simulink model "IEEE9Buses"  (R2024b)
settings: Solver=FixedStepAuto  StartTime=0  StopTime=5  FixedStep=1e-6  RelTol=1e-3
values from neighbouring files (symbols this model uses):
  SG_D_1_D = 0.01056    [SG9_parameters.m]
  SG_D_1_EnableSaturation = 0    [SG9_parameters.m]
  SG_D_1_f0 = 60    [SG9_parameters.m]
  SG_D_1_H = 7.5    [SG9_parameters.m]
  SG_D_1_K_A = 20    [SG9_parameters.m]
  SG_D_1_K_E = 1.000000e+1    (= 10)    [SG9_parameters.m]
  SG_D_1_K_F = 2.363    [SG9_parameters.m]
  SG_D_1_K_s = 5    [SG9_parameters.m]
  SG_D_1_R_a = 0.001088    [SG9_parameters.m]
  SG_D_1_S_A = 1    [SG9_parameters.m]
  SG_D_1_S_B = 0.103    [SG9_parameters.m]
  SG_D_1_S_N = 10.659857    [SG9_parameters.m]
  SG_D_1_SpeedPara = 200    [SG9_parameters.m]
  SG_D_1_T_0 = 0.720173    [SG9_parameters.m]
  SG_D_1_T_1 = 0.3    [SG9_parameters.m]
  SG_D_1_T_2 = 0.05    [SG9_parameters.m]
  SG_D_1_T_3 = 0.02    [SG9_parameters.m]
  SG_D_1_T_4 = 0.005    [SG9_parameters.m]
  SG_D_1_T_A = 0.02    [SG9_parameters.m]
  SG_D_1_T_dd = 8.000000e+0    (= 8)    [SG9_parameters.m]
  SG_D_1_T_ddd = 0.04    [SG9_parameters.m]
  SG_D_1_T_E = 0.314    [SG9_parameters.m]
  SG_D_1_T_F = 0.35    [SG9_parameters.m]
  SG_D_1_T_qd = 0.8    [SG9_parameters.m]
  SG_D_1_T_qdd = 0.02    [SG9_parameters.m]
  SG_D_1_T_speed = 0.1    [SG9_parameters.m]
  SG_D_1_T_w = 0.5    [SG9_parameters.m]
  SG_D_1_V_ref = 1.990276    [SG9_parameters.m]
  SG_D_1_w_ref = 376.991118    [SG9_parameters.m]
  SG_D_1_x_d = 1.9    [SG9_parameters.m]
  SG_D_1_x_dd = 0.302    [SG9_parameters.m]
  SG_D_1_x_ddd = 0.204    [SG9_parameters.m]
  SG_D_1_x_l = 0.05    [SG9_parameters.m]
  SG_D_1_x_q = 1.3    [SG9_parameters.m]
  SG_D_1_x_qd = 0.5    [SG9_parameters.m]
  SG_D_1_x_qdd = 0.3    [SG9_parameters.m]
  SG_D_2_D = 0.01056    [SG9_parameters.m]
  SG_D_2_EnableSaturation = 0    [SG9_parameters.m]
  SG_D_2_f0 = 60    [SG9_parameters.m]
  SG_D_2_H = 7.5    [SG9_parameters.m]
  SG_D_2_K_A = 20    [SG9_parameters.m]
  SG_D_2_K_E = 1.000000e+1    (= 10)    [SG9_parameters.m]
  SG_D_2_K_F = 2.363    [SG9_parameters.m]
  SG_D_2_K_s = 0.5    [SG9_parameters.m]
  SG_D_2_R_a = 0.001088    [SG9_parameters.m]
  SG_D_2_S_A = 1    [SG9_parameters.m]
  SG_D_2_S_B = 0.103    [SG9_parameters.m]
  SG_D_2_S_N = 10.659857    [SG9_parameters.m]
  SG_D_2_SpeedPara = 200    [SG9_parameters.m]
  SG_D_2_T_0 = 1.632913    [SG9_parameters.m]
  SG_D_2_T_1 = 0.2    [SG9_parameters.m]
  SG_D_2_T_2 = 0.05    [SG9_parameters.m]
  SG_D_2_T_3 = 0.02    [SG9_parameters.m]
  SG_D_2_T_4 = 0.005    [SG9_parameters.m]
  SG_D_2_T_A = 0.02    [SG9_parameters.m]
  SG_D_2_T_dd = 8.000000e+0    (= 8)    [SG9_parameters.m]
  SG_D_2_T_ddd = 0.04    [SG9_parameters.m]
  SG_D_2_T_E = 0.314    [SG9_parameters.m]
  SG_D_2_T_F = 0.35    [SG9_parameters.m]
  SG_D_2_T_qd = 0.8    [SG9_parameters.m]
  SG_D_2_T_qdd = 0.02    [SG9_parameters.m]
  SG_D_2_T_speed = 0.1    [SG9_parameters.m]
  SG_D_2_T_w = 0.5    [SG9_parameters.m]
  SG_D_2_V_ref = 2.662631    [SG9_parameters.m]
  SG_D_2_w_ref = 376.991118    [SG9_parameters.m]
  SG_D_2_x_d = 1.9    [SG9_parameters.m]
  SG_D_2_x_dd = 0.302    [SG9_parameters.m]
  SG_D_2_x_ddd = 0.204    [SG9_parameters.m]
  SG_D_2_x_l = 0.05    [SG9_parameters.m]
  SG_D_2_x_q = 1.3    [SG9_parameters.m]
  SG_D_2_x_qd = 0.5    [SG9_parameters.m]
  SG_D_2_x_qdd = 0.3    [SG9_parameters.m]
  SG_D_3_D = 0.01056    [SG9_parameters.m]
  SG_D_3_EnableSaturation = 0    [SG9_parameters.m]
  SG_D_3_f0 = 60    [SG9_parameters.m]
  SG_D_3_H = 7.5    [SG9_parameters.m]
  SG_D_3_K_A = 20    [SG9_parameters.m]
  SG_D_3_K_E = 1.000000e+1    (= 10)    [SG9_parameters.m]
  SG_D_3_K_F = 2.363    [SG9_parameters.m]
  SG_D_3_K_s = 0.5    [SG9_parameters.m]
  SG_D_3_R_a = 0.001088    [SG9_parameters.m]
  SG_D_3_S_A = 1    [SG9_parameters.m]
  SG_D_3_S_B = 0.103    [SG9_parameters.m]
  SG_D_3_S_N = 10.659857    [SG9_parameters.m]
  SG_D_3_SpeedPara = 200    [SG9_parameters.m]
  SG_D_3_T_0 = 0.850788    [SG9_parameters.m]
  SG_D_3_T_1 = 0.2    [SG9_parameters.m]
  SG_D_3_T_2 = 0.05    [SG9_parameters.m]
  SG_D_3_T_3 = 0.02    [SG9_parameters.m]
  SG_D_3_T_4 = 0.005    [SG9_parameters.m]
  SG_D_3_T_A = 0.02    [SG9_parameters.m]
  SG_D_3_T_dd = 8.000000e+0    (= 8)    [SG9_parameters.m]
  SG_D_3_T_ddd = 0.04    [SG9_parameters.m]
  SG_D_3_T_E = 0.314    [SG9_parameters.m]
  SG_D_3_T_F = 0.35    [SG9_parameters.m]
  SG_D_3_T_qd = 0.8    [SG9_parameters.m]
  SG_D_3_T_qdd = 0.02    [SG9_parameters.m]
  SG_D_3_T_speed = 0.1    [SG9_parameters.m]
  SG_D_3_T_w = 0.5    [SG9_parameters.m]
  SG_D_3_V_ref = 1.915682    [SG9_parameters.m]
  SG_D_3_w_ref = 376.991118    [SG9_parameters.m]
  SG_D_3_x_d = 1.9    [SG9_parameters.m]
  SG_D_3_x_dd = 0.302    [SG9_parameters.m]
  SG_D_3_x_ddd = 0.204    [SG9_parameters.m]
  SG_D_3_x_l = 0.05    [SG9_parameters.m]
  SG_D_3_x_q = 1.3    [SG9_parameters.m]
  SG_D_3_x_qd = 0.5    [SG9_parameters.m]
  SG_D_3_x_qdd = 0.3    [SG9_parameters.m]
(part 8 of 9)

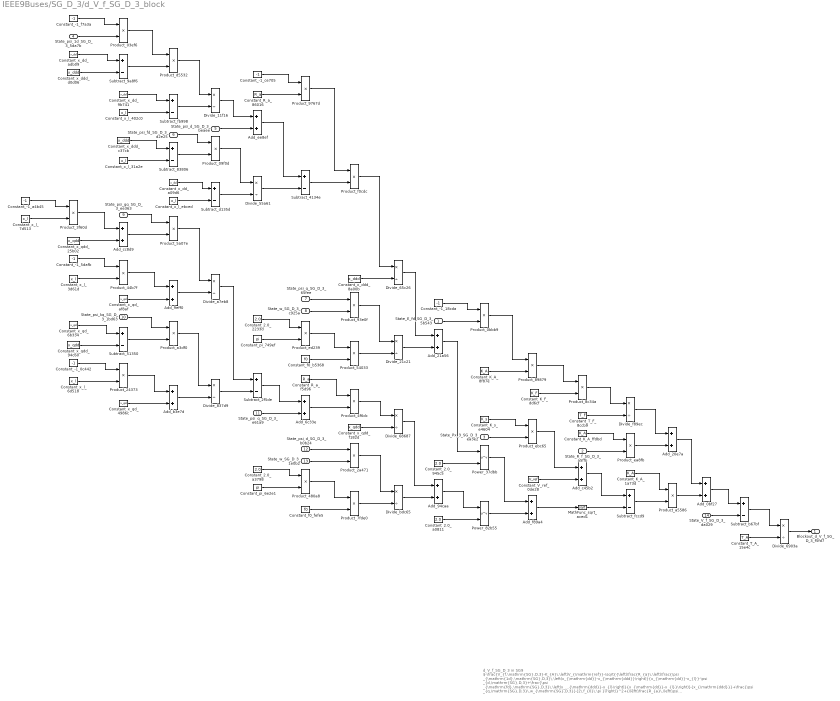
== system IEEE9Buses/SG_D_3/d_V_f_SG_D_3_block ==
  note: d_V_f_SG_D_3 in SG9
      | $-\frac{V_{f,\mathrm{SG},D,3}-K_{A}\,\left(V_{\mathrm{ref}}-\sqrt{{\left(\frac{R_{a}\,\left(\frac{\psi _{\mathrm{1d},\mathrm{SG},D,3}\,\left(x_{\mathrm{dd}}-x_{\mathrm{ddd}}\right)}{x_{\mathrm{dd}}-x_{l}}-\psi _{d,\mathrm{SG},D,3}+\frac{\psi _{\mathrm{fd},\mathrm{SG},D,3}\,\left(x_{\mathrm{ddd}}-x_{l}\right)}{x_{\mathrm{dd}}-x_{l}}\right)}{x_{\mathrm{ddd}}}+\frac{\psi _{q,\mathrm{SG},D,3}\,w_{\mathrm{SG},D,3}}{2\,f_{0}\,\pi }\right)}^2+{\left(\frac{R_{a}\,\left(\psi _{q,\mathrm{SG},D,3}+\frac{\psi _{\mathrm{gq},\mathrm{SG},D,3}\,\left(x_{l}-x_{\mathrm{qdd}}\right)}{x_{l}-x_{\mathrm{qd}}}+\frac{\psi _{\mathrm{kq},\mathrm{SG},D,3}\,\left(x_{\mathrm{qd}}-x_{\mathrm{qdd}}\right)}{x_{l}-x_{\mathrm{qd}}}\right)}{x_{\mathrm{qdd}}}+\frac{\psi _{d,\mathrm{SG},D,3}\,w_{\mathrm{SG},D,3}}{2\,f_{0}\,\pi }\right)}^2}+K_{s}\,\mathrm{Px}_{3,\mathrm{SG},D,3}\right)-K_{A}\,R_{f,\mathrm{SG},D,3}+\frac{E_{\mathrm{fd},\mathrm{SG},D,3}\,K_{A}\,K_{F}}{T_{F}}}{T_{A}}$
      | Automatically generated on 2025-09-12 21:33:42 .
  State_E_fd_SG_D_3_5b543 : Inport
  State_R_f_SG_D_3_a5ffb : Inport  Port=2
  State_Px_3_SG_D_3_ea3e2 : Inport  Port=3
  State_psi_1d_SG_D_3_5da7b : Inport  Port=4
  State_psi_d_SG_D_3_beaee : Inport  Port=5
  State_psi_fd_SG_D_3_d2e25 : Inport  Port=6
  State_psi_q_SG_D_3_65fee : Inport  Port=7
  State_w_SG_D_3_c925a : Inport  Port=8
  State_psi_gq_SG_D_3_ee363 : Inport  Port=9
  State_psi_kq_SG_D_3_1bd63 : Inport  Port=10
  State_psi_q_SG_D_3_e61a9 : Inport  Port=11
  State_psi_d_SG_D_3_b0b24 : Inport  Port=12
  State_w_SG_D_3_1e0b2 : Inport  Port=13
  State_V_f_SG_D_3_da029 : Inport  Port=14
  Add_0bf27 : Sum
  Add_20e7a : Sum
  Add_21a56 : Sum
  Add_6c33e : Sum
  Add_94caa : Sum
  Add_9eff0 : Sum
  Add_b3e7d : Sum
  Add_c45b2 : Sum
  Add_cc8d9 : Sum
  Add_ee8ef : Sum
  Add_f89a4 : Sum
  Constant_-1_0c442 : Constant  Value=-1
  Constant_-1_18cda : Constant  Value=-1
  Constant_-1_5dafb : Constant  Value=-1
  Constant_-1_a4b45 : Constant  Value=-1
  Constant_-1_ce705 : Constant  Value=-1
  Constant_-1_f7a3a : Constant  Value=-1
  Constant_2.0_2233d : Constant  Value=2.0
  Constant_2.0_945c5 : Constant  Value=2.0
  Constant_2.0_a0811 : Constant  Value=2.0
  Constant_2.0_a3798 : Constant  Value=2.0
  Constant_K_A_1a73d : Constant  Value=K_A
  Constant_K_A_8f87e : Constant  Value=K_A
  Constant_K_A_ffdbd : Constant  Value=K_A
  Constant_K_F_dd6cf : Constant  Value=K_F
  Constant_K_s_e4604 : Constant  Value=K_s
  Constant_R_a_86016 : Constant  Value=R_a
  Constant_R_a_f5d96 : Constant  Value=R_a
  Constant_T_A_15e4c : Constant  Value=T_A
  Constant_T_F_8ccb9 : Constant  Value=T_F
  Constant_V_ref_0de28 : Constant  Value=V_ref
  Constant_f0_b5368 : Constant  Value=f0
  Constant_f0_fefe5 : Constant  Value=f0
  Constant_pi_6e2e1 : Constant  Value=pi
  Constant_pi_749ef : Constant  Value=pi
  Constant_x_dd_9b741 : Constant  Value=x_dd
  Constant_x_dd_a09d6 : Constant  Value=x_dd
  Constant_x_dd_adb09 : Constant  Value=x_dd
  Constant_x_ddd_8a00b : Constant  Value=x_ddd
  Constant_x_ddd_c37cb : Constant  Value=x_ddd
  Constant_x_ddd_d0d06 : Constant  Value=x_ddd
  Constant_x_l_31a2e : Constant  Value=x_l
  Constant_x_l_3d61d : Constant  Value=x_l
  Constant_x_l_402c0 : Constant  Value=x_l
  Constant_x_l_6d518 : Constant  Value=x_l
  Constant_x_l_7d513 : Constant  Value=x_l
  Constant_x_l_ebced : Constant  Value=x_l
  Constant_x_qd_4986c : Constant  Value=x_qd
  Constant_x_qd_6b334 : Constant  Value=x_qd
  Constant_x_qd_af8af : Constant  Value=x_qd
  Constant_x_qdd_25b02 : Constant  Value=x_qdd
  Constant_x_qdd_94c60 : Constant  Value=x_qdd
  Constant_x_qdd_f182d : Constant  Value=x_qdd
  Divide_11f16 : Product  Inputs=*/
  Divide_21c21 : Product  Inputs=*/
  Divide_55a61 : Product  Inputs=*/
  Divide_65c26 : Product  Inputs=*/
  Divide_68687 : Product  Inputs=*/
  Divide_6903a : Product  Inputs=*/
  Divide_837d9 : Product  Inputs=*/
  Divide_a7eb8 : Product  Inputs=*/
  Divide_bdc65 : Product  Inputs=*/
  Divide_f89ec : Product  Inputs=*/
  MathFunc_sqrt_aced1 : Sqrt
  Power_37dbb : Math  Operator=pow
  Power_82b55 : Math  Operator=pow
  Product_03ef6 : Product
  Product_09f0d : Product
  Product_0bbb9 : Product
  Product_24373 : Product
  Product_2a471 : Product
  Product_3f60d : Product
  Product_44b7f : Product
  Product_480a8 : Product
  Product_4f6dc : Product
  Product_54033 : Product
  Product_5a07e : Product
  Product_7fde0 : Product
  Product_89879 : Product
  Product_8c34a : Product
  Product_93e0f : Product
  Product_9767d : Product
  Product_a3df0 : Product
  Product_a5586 : Product
  Product_d5532 : Product
  Product_ea8fb : Product
  Product_ebc65 : Product
  Product_ed239 : Product
  Product_f0cdc : Product
  Subtract_2f5de : Sum  Inputs=+-
  Subtract_4134e : Sum  Inputs=+-
  Subtract_51350 : Sum  Inputs=+-
  Subtract_83806 : Sum  Inputs=+-
  Subtract_9a8f6 : Sum  Inputs=+-
  Subtract_b67bf : Sum  Inputs=+-
  Subtract_d135d : Sum  Inputs=+-
  Subtract_fb998 : Sum  Inputs=+-
  Subtract_fccd9 : Sum  Inputs=+-
  Blockout_d_V_f_SG_D_3_f5fd7 : Outport
  wires:
  Constant_K_A_ffdbd/1 -> Product_ea8fb/1
  Constant_-1_a4b45/1 -> Product_3f60d/1
  Subtract_83806/1 -> Product_09f0d/2
  Constant_x_l_7d513/1 -> Product_3f60d/2
  Divide_bdc65/1 -> Add_94caa/2
  Constant_-1_f7a3a/1 -> Product_03ef6/1
  State_psi_1d_SG_D_3_5da7b/1 -> Product_03ef6/2
  Constant_x_dd_adb09/1 -> Subtract_9a8f6/1
  Divide_55a61/1 -> Subtract_4134e/2
  Product_3f60d/1 -> Add_cc8d9/1
  Constant_x_qdd_25b02/1 -> Add_cc8d9/2
  Constant_x_ddd_d0d06/1 -> Subtract_9a8f6/2
  Constant_2.0_a0811/1 -> Power_82b55/2
  Constant_-1_5dafb/1 -> Product_44b7f/1
  Divide_a7eb8/1 -> Subtract_2f5de/1
  Subtract_fb998/1 -> Divide_11f16/2
  Constant_x_l_3d61d/1 -> Product_44b7f/2
  Constant_x_qd_6b334/1 -> Subtract_51350/1
  State_w_SG_D_3_c925a/1 -> Product_93e0f/2
  Constant_x_qdd_94c60/1 -> Subtract_51350/2
  Constant_2.0_2233d/1 -> Product_ed239/1
  Constant_-1_0c442/1 -> Product_24373/1
  Constant_pi_749ef/1 -> Product_ed239/2
  Add_ee8ef/1 -> Subtract_4134e/1
  Constant_x_l_6d518/1 -> Product_24373/2
  Product_03ef6/1 -> Product_d5532/1
  Subtract_9a8f6/1 -> Product_d5532/2
  Constant_2.0_a3798/1 -> Product_480a8/1
  Constant_x_dd_9b741/1 -> Subtract_fb998/1
  Constant_pi_6e2e1/1 -> Product_480a8/2
  Constant_x_l_402c0/1 -> Subtract_fb998/2
  Constant_x_ddd_c37cb/1 -> Subtract_83806/1
  Constant_x_l_31a2e/1 -> Subtract_83806/2
  State_psi_gq_SG_D_3_ee363/1 -> Product_5a07e/1
  Constant_x_l_ebced/1 -> Subtract_d135d/2
  Add_cc8d9/1 -> Product_5a07e/2
  Product_44b7f/1 -> Add_9eff0/1
  Product_5a07e/1 -> Divide_a7eb8/1
  Constant_x_qd_af8af/1 -> Add_9eff0/2
  State_psi_kq_SG_D_3_1bd63/1 -> Product_a3df0/1
  State_psi_q_SG_D_3_65fee/1 -> Product_93e0f/1
  Add_21a56/1 -> Power_37dbb/1
  Subtract_51350/1 -> Product_a3df0/2
  Constant_f0_b5368/1 -> Product_54033/2
  Product_ed239/1 -> Product_54033/1
  Constant_x_qd_4986c/1 -> Add_b3e7d/2
  Product_24373/1 -> Add_b3e7d/1
  Product_d5532/1 -> Divide_11f16/1
  State_psi_fd_SG_D_3_d2e25/1 -> Product_09f0d/1
  Constant_x_dd_a09d6/1 -> Subtract_d135d/1
  Add_9eff0/1 -> Divide_a7eb8/2
  Add_f89a4/1 -> MathFunc_sqrt_aced1/1
  Product_a3df0/1 -> Divide_837d9/1
  Add_b3e7d/1 -> Divide_837d9/2
  Product_9767d/1 -> Product_f0cdc/1
  Divide_11f16/1 -> Add_ee8ef/1
  Add_c45b2/1 -> Subtract_fccd9/1
  State_psi_d_SG_D_3_beaee/1 -> Add_ee8ef/2
  Product_09f0d/1 -> Divide_55a61/1
  Subtract_d135d/1 -> Divide_55a61/2
  MathFunc_sqrt_aced1/1 -> Subtract_fccd9/2
  Divide_837d9/1 -> Subtract_2f5de/2
  Constant_-1_ce705/1 -> Product_9767d/1
  Constant_R_a_86016/1 -> Product_9767d/2
  Subtract_2f5de/1 -> Add_6c33e/1
  State_psi_q_SG_D_3_e61a9/1 -> Add_6c33e/2
  Subtract_4134e/1 -> Product_f0cdc/2
  Constant_R_a_f5d96/1 -> Product_4f6dc/1
  Add_6c33e/1 -> Product_4f6dc/2
  State_psi_d_SG_D_3_b0b24/1 -> Product_2a471/1
  State_w_SG_D_3_1e0b2/1 -> Product_2a471/2
  Product_480a8/1 -> Product_7fde0/1
  Constant_f0_fefe5/1 -> Product_7fde0/2
  Product_f0cdc/1 -> Divide_65c26/1
  Constant_x_ddd_8a00b/1 -> Divide_65c26/2
  Product_93e0f/1 -> Divide_21c21/1
  Product_54033/1 -> Divide_21c21/2
  Product_4f6dc/1 -> Divide_68687/1
  Constant_x_qdd_f182d/1 -> Divide_68687/2
  Product_2a471/1 -> Divide_bdc65/1
  Product_7fde0/1 -> Divide_bdc65/2
  Divide_65c26/1 -> Add_21a56/1
  Divide_21c21/1 -> Add_21a56/2
  Divide_68687/1 -> Add_94caa/1
  Constant_-1_18cda/1 -> Product_0bbb9/1
  State_E_fd_SG_D_3_5b543/1 -> Product_0bbb9/2
  Constant_2.0_945c5/1 -> Power_37dbb/2
  Add_94caa/1 -> Power_82b55/1
  Product_0bbb9/1 -> Product_89879/1
  Constant_K_A_8f87e/1 -> Product_89879/2
  Constant_K_s_e4604/1 -> Product_ebc65/1
  State_Px_3_SG_D_3_ea3e2/1 -> Product_ebc65/2
  Power_37dbb/1 -> Add_f89a4/1
  Power_82b55/1 -> Add_f89a4/2
  Product_89879/1 -> Product_8c34a/1
  Constant_K_F_dd6cf/1 -> Product_8c34a/2
  Product_ebc65/1 -> Add_c45b2/1
  Constant_V_ref_0de28/1 -> Add_c45b2/2
  Product_8c34a/1 -> Divide_f89ec/1
  Constant_T_F_8ccb9/1 -> Divide_f89ec/2
  Add_0bf27/1 -> Subtract_b67bf/1
  State_R_f_SG_D_3_a5ffb/1 -> Product_ea8fb/2
  Divide_f89ec/1 -> Add_20e7a/1
  Product_ea8fb/1 -> Add_20e7a/2
  Constant_K_A_1a73d/1 -> Product_a5586/1
  Subtract_fccd9/1 -> Product_a5586/2
  Add_20e7a/1 -> Add_0bf27/1
  Product_a5586/1 -> Add_0bf27/2
  State_V_f_SG_D_3_da029/1 -> Subtract_b67bf/2
  Subtract_b67bf/1 -> Divide_6903a/1
  Constant_T_A_15e4c/1 -> Divide_6903a/2
  Divide_6903a/1 -> Blockout_d_V_f_SG_D_3_f5fd7/1

== system IEEE9Buses/SG_D_3/d_psi_1d_SG_D_3_block ==
  note: d_psi_1d_SG_D_3 in SG9
      | $-\frac{\psi _{\mathrm{1d},\mathrm{SG},D,3}-\psi _{\mathrm{fd},\mathrm{SG},D,3}+\frac{\left(x_{\mathrm{dd}}-x_{l}\right)\,\left(\frac{\psi _{\mathrm{1d},\mathrm{SG},D,3}\,\left(x_{\mathrm{dd}}-x_{\mathrm{ddd}}\right)}{x_{\mathrm{dd}}-x_{l}}-\psi _{d,\mathrm{SG},D,3}+\frac{\psi _{\mathrm{fd},\mathrm{SG},D,3}\,\left(x_{\mathrm{ddd}}-x_{l}\right)}{x_{\mathrm{dd}}-x_{l}}\right)}{x_{\mathrm{ddd}}}}{T_{\mathrm{ddd}}}$
      | Automatically generated on 2025-09-12 21:33:17 .
  State_psi_1d_SG_D_3_400ff : Inport
  State_psi_fd_SG_D_3_31a8d : Inport  Port=2
  State_psi_1d_SG_D_3_f2eaa : Inport  Port=3
  State_psi_d_SG_D_3_c9b51 : Inport  Port=4
  State_psi_fd_SG_D_3_47081 : Inport  Port=5
  Add_42e95 : Sum
  Add_4c52e : Sum
  Add_9e772 : Sum
  Constant_-1_54a57 : Constant  Value=-1
  Constant_-1_6696c : Constant  Value=-1
  Constant_T_ddd_7d9a7 : Constant  Value=T_ddd
  Constant_x_dd_313f0 : Constant  Value=x_dd
  Constant_x_dd_447e3 : Constant  Value=x_dd
  Constant_x_dd_5a1d4 : Constant  Value=x_dd
  Constant_x_dd_6452b : Constant  Value=x_dd
  Constant_x_ddd_d782d : Constant  Value=x_ddd
  Constant_x_ddd_f181f : Constant  Value=x_ddd
  Constant_x_ddd_f90f1 : Constant  Value=x_ddd
  Constant_x_l_03c08 : Constant  Value=x_l
  Constant_x_l_57332 : Constant  Value=x_l
  Constant_x_l_6982e : Constant  Value=x_l
  Constant_x_l_f8376 : Constant  Value=x_l
  Divide_209ea : Product  Inputs=*/
  Divide_21392 : Product  Inputs=*/
  Divide_56b1a : Product  Inputs=*/
  Divide_59c36 : Product  Inputs=*/
  Product_2f78e : Product
  Product_628a4 : Product
  Product_9daab : Product
  Product_a8839 : Product
  Product_cc23d : Product
  Subtract_222c1 : Sum  Inputs=+-
  Subtract_2de3d : Sum  Inputs=+-
  Subtract_d21cf : Sum  Inputs=+-
  Subtract_d485e : Sum  Inputs=+-
  Subtract_d4c0d : Sum  Inputs=+-
  Subtract_f157f : Sum  Inputs=+-
  Blockout_d_psi_1d_SG_D_3_883d4 : Outport
  wires:
  Divide_59c36/1 -> Add_4c52e/1
  Subtract_222c1/1 -> Product_a8839/2
  Constant_-1_54a57/1 -> Product_9daab/1
  Constant_x_dd_5a1d4/1 -> Subtract_d4c0d/1
  State_psi_1d_SG_D_3_f2eaa/1 -> Product_9daab/2
  Product_9daab/1 -> Product_a8839/1
  Constant_x_dd_447e3/1 -> Subtract_222c1/1
  Constant_x_ddd_f90f1/1 -> Subtract_222c1/2
  Constant_x_l_6982e/1 -> Subtract_d4c0d/2
  Constant_x_ddd_d782d/1 -> Subtract_d485e/1
  Divide_209ea/1 -> Blockout_d_psi_1d_SG_D_3_883d4/1
  Constant_x_l_57332/1 -> Subtract_d485e/2
  Product_a8839/1 -> Divide_59c36/1
  Subtract_d4c0d/1 -> Divide_59c36/2
  State_psi_fd_SG_D_3_47081/1 -> Product_2f78e/1
  Subtract_d485e/1 -> Product_2f78e/2
  Constant_x_dd_313f0/1 -> Subtract_d21cf/1
  Constant_x_l_03c08/1 -> Subtract_d21cf/2
  State_psi_d_SG_D_3_c9b51/1 -> Add_4c52e/2
  Product_2f78e/1 -> Divide_21392/1
  Subtract_d21cf/1 -> Divide_21392/2
  Constant_x_dd_6452b/1 -> Subtract_f157f/1
  Constant_x_l_f8376/1 -> Subtract_f157f/2
  Add_4c52e/1 -> Subtract_2de3d/1
  Divide_21392/1 -> Subtract_2de3d/2
  Constant_-1_6696c/1 -> Product_628a4/1
  State_psi_1d_SG_D_3_400ff/1 -> Product_628a4/2
  State_psi_fd_SG_D_3_31a8d/1 -> Add_42e95/2
  Subtract_f157f/1 -> Product_cc23d/1
  Subtract_2de3d/1 -> Product_cc23d/2
  Product_628a4/1 -> Add_42e95/1
  Product_cc23d/1 -> Divide_56b1a/1
  Constant_x_ddd_f181f/1 -> Divide_56b1a/2
  Add_42e95/1 -> Add_9e772/1
  Divide_56b1a/1 -> Add_9e772/2
  Add_9e772/1 -> Divide_209ea/1
  Constant_T_ddd_7d9a7/1 -> Divide_209ea/2

== system IEEE9Buses/SG_D_3/d_psi_d_SG_D_3_block ==
  note: d_psi_d_SG_D_3 in SG9
      | $2\,\pi \,f_{0}\,\left(v_{d,\mathrm{SG},D,3}\,\sin\left(\theta _{\mathrm{SG},D,3}\right)-v_{q,\mathrm{SG},D,3}\,\cos\left(\theta _{\mathrm{SG},D,3}\right)+\frac{R_{a}\,\left(\frac{\psi _{\mathrm{1d},\mathrm{SG},D,3}\,\left(x_{\mathrm{dd}}-x_{\mathrm{ddd}}\right)}{x_{\mathrm{dd}}-x_{l}}-\psi _{d,\mathrm{SG},D,3}+\frac{\psi _{\mathrm{fd},\mathrm{SG},D,3}\,\left(x_{\mathrm{ddd}}-x_{l}\right)}{x_{\mathrm{dd}}-x_{l}}\right)}{x_{\mathrm{ddd}}}+\frac{\psi _{q,\mathrm{SG},D,3}\,w_{\mathrm{SG},D,3}}{2\,f_{0}\,\pi }\right)$
      | Automatically generated on 2025-09-12 21:33:05 .
  State_psi_1d_SG_D_3_df20d : Inport
  State_psi_d_SG_D_3_5cf2c : Inport  Port=2
  State_psi_fd_SG_D_3_e8974 : Inport  Port=3
  Input_v_d_SG_D_3_a409b : Inport  Port=4
  State_theta_SG_D_3_fa0de : Inport  Port=5
  Input_v_q_SG_D_3_73a19 : Inport  Port=6
  State_theta_SG_D_3_450d2 : Inport  Port=7
  State_psi_q_SG_D_3_3cdee : Inport  Port=8
  State_w_SG_D_3_3c685 : Inport  Port=9
  Add_4bd27 : Sum
  Add_a9d77 : Sum
  Constant_-1_956ee : Constant  Value=-1
  Constant_-2.0_730ca : Constant  Value=-2.0
  Constant_2.0_7512b : Constant  Value=2.0
  Constant_R_a_2c184 : Constant  Value=R_a
  Constant_f0_5f857 : Constant  Value=f0
  Constant_f0_a215f : Constant  Value=f0
  Constant_pi_2d0c1 : Constant  Value=pi
  Constant_pi_a1e68 : Constant  Value=pi
  Constant_x_dd_29953 : Constant  Value=x_dd
  Constant_x_dd_be334 : Constant  Value=x_dd
  Constant_x_dd_bf9bd : Constant  Value=x_dd
  Constant_x_ddd_58709 : Constant  Value=x_ddd
  Constant_x_ddd_84af1 : Constant  Value=x_ddd
  Constant_x_ddd_f35e7 : Constant  Value=x_ddd
  Constant_x_l_06f8d : Constant  Value=x_l
  Constant_x_l_781b5 : Constant  Value=x_l
  Constant_x_l_81dc9 : Constant  Value=x_l
  Divide_3a0c2 : Product  Inputs=*/
  Divide_8a45c : Product  Inputs=*/
  Divide_eab3b : Product  Inputs=*/
  Divide_fffea : Product  Inputs=*/
  MathFunc_cos_6cb2b : Trigonometry  Operator=cos
  MathFunc_sin_c609b : Trigonometry
  Product_075f4 : Product
  Product_1f547 : Product
  Product_53eb6 : Product
  Product_5c8ff : Product
  Product_865d8 : Product
  Product_8be05 : Product
  Product_a313a : Product
  Product_a5a4e : Product
  Product_bb93c : Product
  Product_cddda : Product
  Product_e0659 : Product
  Product_eda06 : Product
  Subtract_46059 : Sum  Inputs=+-
  Subtract_672d9 : Sum  Inputs=+-
  Subtract_6feec : Sum  Inputs=+-
  Subtract_76533 : Sum  Inputs=+-
  Subtract_9ad1c : Sum  Inputs=+-
  Subtract_9d906 : Sum  Inputs=+-
  Subtract_f1390 : Sum  Inputs=+-
  Blockout_d_psi_d_SG_D_3_6cd1a : Outport
  wires:
  Constant_-1_956ee/1 -> Product_a313a/1
  Constant_2.0_7512b/1 -> Product_865d8/1
  Constant_x_dd_bf9bd/1 -> Subtract_f1390/1
  State_psi_1d_SG_D_3_df20d/1 -> Product_a313a/2
  Constant_x_dd_be334/1 -> Subtract_9d906/1
  Constant_pi_a1e68/1 -> Product_865d8/2
  Constant_x_ddd_84af1/1 -> Subtract_f1390/2
  Product_a313a/1 -> Product_e0659/1
  Product_865d8/1 -> Product_8be05/1
  Subtract_f1390/1 -> Product_e0659/2
  Constant_-2.0_730ca/1 -> Product_eda06/1
  Constant_x_l_06f8d/1 -> Subtract_9d906/2
  Constant_x_ddd_58709/1 -> Subtract_9ad1c/1
  Constant_pi_2d0c1/1 -> Product_eda06/2
  Constant_x_l_781b5/1 -> Subtract_9ad1c/2
  Product_bb93c/1 -> Divide_8a45c/1
  Product_e0659/1 -> Divide_fffea/1
  Subtract_9d906/1 -> Divide_fffea/2
  State_psi_fd_SG_D_3_e8974/1 -> Product_5c8ff/1
  Subtract_9ad1c/1 -> Product_5c8ff/2
  Constant_x_dd_29953/1 -> Subtract_46059/1
  Constant_x_l_81dc9/1 -> Subtract_46059/2
  Divide_8a45c/1 -> Subtract_672d9/2
  Divide_fffea/1 -> Add_4bd27/1
  Subtract_6feec/1 -> Product_075f4/2
  State_psi_d_SG_D_3_5cf2c/1 -> Add_4bd27/2
  Product_5c8ff/1 -> Divide_eab3b/1
  Subtract_46059/1 -> Divide_eab3b/2
  Add_4bd27/1 -> Subtract_6feec/1
  Divide_eab3b/1 -> Subtract_6feec/2
  Product_a5a4e/1 -> Add_a9d77/2
  Constant_R_a_2c184/1 -> Product_075f4/1
  Product_53eb6/1 -> Product_cddda/1
  State_theta_SG_D_3_fa0de/1 -> MathFunc_sin_c609b/1
  Product_075f4/1 -> Divide_3a0c2/1
  Constant_x_ddd_f35e7/1 -> Divide_3a0c2/2
  Input_v_d_SG_D_3_a409b/1 -> Product_1f547/1
  State_w_SG_D_3_3c685/1 -> Product_bb93c/2
  MathFunc_sin_c609b/1 -> Product_1f547/2
  State_theta_SG_D_3_450d2/1 -> MathFunc_cos_6cb2b/1
  MathFunc_cos_6cb2b/1 -> Product_a5a4e/2
  Divide_3a0c2/1 -> Subtract_76533/1
  Product_1f547/1 -> Subtract_76533/2
  Input_v_q_SG_D_3_73a19/1 -> Product_a5a4e/1
  State_psi_q_SG_D_3_3cdee/1 -> Product_bb93c/1
  Constant_f0_a215f/1 -> Product_8be05/2
  Subtract_76533/1 -> Add_a9d77/1
  Product_8be05/1 -> Divide_8a45c/2
  Product_eda06/1 -> Product_53eb6/1
  Constant_f0_5f857/1 -> Product_53eb6/2
  Add_a9d77/1 -> Subtract_672d9/1
  Subtract_672d9/1 -> Product_cddda/2
  Product_cddda/1 -> Blockout_d_psi_d_SG_D_3_6cd1a/1

== system IEEE9Buses/SG_D_3/d_psi_fd_SG_D_3_block ==
  note: d_psi_fd_SG_D_3 in SG9
      | $-\frac{\psi _{\mathrm{fd},\mathrm{SG},D,3}-E_{\mathrm{fd},\mathrm{SG},D,3}+\left(x_{d}-x_{\mathrm{dd}}\right)\,\left(\frac{\frac{\psi _{\mathrm{1d},\mathrm{SG},D,3}\,\left(x_{\mathrm{dd}}-x_{\mathrm{ddd}}\right)}{x_{\mathrm{dd}}-x_{l}}-\psi _{d,\mathrm{SG},D,3}+\frac{\psi _{\mathrm{fd},\mathrm{SG},D,3}\,\left(x_{\mathrm{ddd}}-x_{l}\right)}{x_{\mathrm{dd}}-x_{l}}}{x_{\mathrm{ddd}}}-\frac{\left(x_{\mathrm{dd}}-x_{\mathrm{ddd}}\right)\,\left(\psi _{\mathrm{1d},\mathrm{SG},D,3}-\psi _{\mathrm{fd},\mathrm{SG},D,3}+\frac{\left(x_{\mathrm{dd}}-x_{l}\right)\,\left(\frac{\psi _{\mathrm{1d},\mathrm{SG},D,3}\,\left(x_{\mathrm{dd}}-x_{\mathrm{ddd}}\right)}{x_{\mathrm{dd}}-x_{l}}-\psi _{d,\mathrm{SG},D,3}+\frac{\psi _{\mathrm{fd},\mathrm{SG},D,3}\,\left(x_{\mathrm{ddd}}-x_{l}\right)}{x_{\mathrm{dd}}-x_{l}}\right)}{x_{\mathrm{ddd}}}\right)}{{\left(x_{\mathrm{dd}}-x_{l}\right)}^2}\right)}{T_{\mathrm{dd}}}$
      | Automatically generated on 2025-09-12 21:33:14 .
  State_E_fd_SG_D_3_2d5b6 : Inport
  State_psi_fd_SG_D_3_8c274 : Inport  Port=2
  State_psi_1d_SG_D_3_ced24 : Inport  Port=3
  State_psi_fd_SG_D_3_4a37b : Inport  Port=4
  State_psi_1d_SG_D_3_58f7d : Inport  Port=5
  State_psi_d_SG_D_3_264cd : Inport  Port=6
  State_psi_fd_SG_D_3_d3958 : Inport  Port=7
  State_psi_1d_SG_D_3_6cc6d : Inport  Port=8
  State_psi_d_SG_D_3_3305b : Inport  Port=9
  State_psi_fd_SG_D_3_265a7 : Inport  Port=10
  Add_315d4 : Sum
  Add_a78bb : Sum
  Constant_-1_2d1a2 : Constant  Value=-1
  Constant_-1_a4354 : Constant  Value=-1
  Constant_-1_b314b : Constant  Value=-1
  Constant_2.0_a7a8d : Constant  Value=2.0
  Constant_T_dd_9c02c : Constant  Value=T_dd
  Constant_x_d_df3b7 : Constant  Value=x_d
  Constant_x_dd_05d1b : Constant  Value=x_dd
  Constant_x_dd_0c92f : Constant  Value=x_dd
  Constant_x_dd_15bda : Constant  Value=x_dd
  Constant_x_dd_2465f : Constant  Value=x_dd
  Constant_x_dd_5b54a : Constant  Value=x_dd
  Constant_x_dd_8d7a4 : Constant  Value=x_dd
  Constant_x_dd_a5419 : Constant  Value=x_dd
  Constant_x_dd_daca3 : Constant  Value=x_dd
  Constant_x_dd_e1b8f : Constant  Value=x_dd
  Constant_x_dd_ee6c4 : Constant  Value=x_dd
  Constant_x_ddd_4286f : Constant  Value=x_ddd
  Constant_x_ddd_71c11 : Constant  Value=x_ddd
  Constant_x_ddd_a541b : Constant  Value=x_ddd
  Constant_x_ddd_b4a45 : Constant  Value=x_ddd
  Constant_x_ddd_dc6f5 : Constant  Value=x_ddd
  Constant_x_ddd_df8f7 : Constant  Value=x_ddd
  Constant_x_ddd_e0756 : Constant  Value=x_ddd
  Constant_x_l_1a534 : Constant  Value=x_l
  Constant_x_l_1f6b0 : Constant  Value=x_l
  Constant_x_l_2b5b1 : Constant  Value=x_l
  Constant_x_l_4829f : Constant  Value=x_l
  Constant_x_l_7086f : Constant  Value=x_l
  Constant_x_l_a8aaa : Constant  Value=x_l
  Constant_x_l_c667f : Constant  Value=x_l
  Constant_x_l_e9b20 : Constant  Value=x_l
  Divide_02eba : Product  Inputs=*/
  Divide_1a77f : Product  Inputs=*/
  Divide_27c8b : Product  Inputs=*/
  Divide_b6dbe : Product  Inputs=*/
  Divide_d6283 : Product  Inputs=*/
  Divide_d8b78 : Product  Inputs=*/
  Divide_dcd7a : Product  Inputs=*/
  Divide_fc87f : Product  Inputs=*/
  Power_48757 : Math  Operator=pow
  Product_11951 : Product
  Product_1752c : Product
  Product_2d1c1 : Product
  Product_46251 : Product
  Product_6386e : Product
  Product_8257a : Product
  Product_d12fa : Product
  Product_f68fa : Product
  Product_f8d33 : Product
  Product_f9dbb : Product
  Subtract_00c84 : Sum  Inputs=+-
  Subtract_05aad : Sum  Inputs=+-
  Subtract_07df4 : Sum  Inputs=+-
  Subtract_0afce : Sum  Inputs=+-
  Subtract_1063e : Sum  Inputs=+-
  Subtract_19629 : Sum  Inputs=+-
  Subtract_1984b : Sum  Inputs=+-
  Subtract_1aa7b : Sum  Inputs=+-
  Subtract_1da0a : Sum  Inputs=+-
  Subtract_34b29 : Sum  Inputs=+-
  Subtract_3c84b : Sum  Inputs=+-
  Subtract_617ae : Sum  Inputs=+-
  Subtract_6e185 : Sum  Inputs=+-
  Subtract_71270 : Sum  Inputs=+-
  Subtract_8e9e6 : Sum  Inputs=+-
  Subtract_b7431 : Sum  Inputs=+-
  Subtract_debb7 : Sum  Inputs=+-
  Subtract_f7d48 : Sum  Inputs=+-
  Subtract_fb39e : Sum  Inputs=+-
  Blockout_d_psi_fd_SG_D_3_c1dbd : Outport
  wires:
  Product_f9dbb/1 -> Divide_1a77f/1
  Constant_-1_a4354/1 -> Product_2d1c1/1
  Subtract_07df4/1 -> Product_8257a/2
  State_psi_1d_SG_D_3_58f7d/1 -> Product_2d1c1/2
  Constant_x_l_e9b20/1 -> Subtract_1da0a/2
  Constant_x_dd_5b54a/1 -> Subtract_07df4/1
  Constant_x_ddd_4286f/1 -> Subtract_07df4/2
  Product_2d1c1/1 -> Product_8257a/1
  Constant_x_dd_15bda/1 -> Subtract_f7d48/1
  Constant_x_l_2b5b1/1 -> Subtract_f7d48/2
  Constant_x_ddd_dc6f5/1 -> Subtract_05aad/2
  Constant_x_ddd_71c11/1 -> Subtract_1984b/1
  Constant_x_l_c667f/1 -> Subtract_1984b/2
  Product_46251/1 -> Product_1752c/1
  Product_8257a/1 -> Divide_d6283/1
  Subtract_f7d48/1 -> Divide_d6283/2
  State_psi_fd_SG_D_3_d3958/1 -> Product_6386e/1
  Constant_x_ddd_df8f7/1 -> Subtract_1da0a/1
  Subtract_1984b/1 -> Product_6386e/2
  Constant_x_dd_a5419/1 -> Subtract_fb39e/1
  Constant_-1_2d1a2/1 -> Product_46251/1
  Constant_x_l_4829f/1 -> Subtract_fb39e/2
  Product_1752c/1 -> Divide_02eba/1
  Divide_d6283/1 -> Add_a78bb/1
  Product_d12fa/1 -> Divide_d8b78/1
  State_psi_d_SG_D_3_264cd/1 -> Add_a78bb/2
  State_psi_fd_SG_D_3_265a7/1 -> Product_d12fa/1
  Product_6386e/1 -> Divide_fc87f/1
  Constant_x_dd_05d1b/1 -> Subtract_b7431/1
  Subtract_fb39e/1 -> Divide_fc87f/2
  Constant_x_l_1f6b0/1 -> Subtract_34b29/2
  Constant_x_dd_2465f/1 -> Subtract_3c84b/1
  Subtract_8e9e6/1 -> Product_f68fa/2
  Constant_x_l_a8aaa/1 -> Subtract_3c84b/2
  Divide_02eba/1 -> Add_315d4/1
  Constant_x_ddd_b4a45/1 -> Divide_1a77f/2
  Add_a78bb/1 -> Subtract_71270/1
  Divide_fc87f/1 -> Subtract_71270/2
  State_psi_1d_SG_D_3_6cc6d/1 -> Product_46251/2
  Constant_x_l_1a534/1 -> Subtract_b7431/2
  Constant_x_dd_daca3/1 -> Subtract_05aad/1
  Subtract_3c84b/1 -> Product_f9dbb/1
  Add_315d4/1 -> Subtract_debb7/1
  Subtract_71270/1 -> Product_f9dbb/2
  Subtract_05aad/1 -> Product_1752c/2
  Constant_x_dd_ee6c4/1 -> Subtract_1aa7b/1
  Constant_x_l_7086f/1 -> Subtract_1aa7b/2
  Subtract_1da0a/1 -> Product_d12fa/2
  Constant_x_dd_0c92f/1 -> Subtract_8e9e6/1
  Constant_x_ddd_e0756/1 -> Subtract_8e9e6/2
  Product_f68fa/1 -> Product_f8d33/1
  State_psi_1d_SG_D_3_ced24/1 -> Subtract_00c84/1
  Subtract_1aa7b/1 -> Divide_02eba/2
  State_psi_fd_SG_D_3_4a37b/1 -> Subtract_00c84/2
  Constant_-1_b314b/1 -> Product_f68fa/1
  Subtract_00c84/1 -> Subtract_6e185/1
  Divide_1a77f/1 -> Subtract_6e185/2
  Constant_x_dd_e1b8f/1 -> Subtract_34b29/1
  Divide_d8b78/1 -> Subtract_debb7/2
  State_psi_d_SG_D_3_3305b/1 -> Add_315d4/2
  Subtract_b7431/1 -> Divide_d8b78/2
  Subtract_6e185/1 -> Product_f8d33/2
  Subtract_34b29/1 -> Power_48757/1
  Constant_2.0_a7a8d/1 -> Power_48757/2
  Product_f8d33/1 -> Divide_dcd7a/1
  Subtract_0afce/1 -> Product_11951/2
  Power_48757/1 -> Divide_dcd7a/2
  Subtract_debb7/1 -> Divide_b6dbe/1
  Constant_x_ddd_a541b/1 -> Divide_b6dbe/2
  Constant_x_d_df3b7/1 -> Subtract_1063e/1
  Constant_x_dd_8d7a4/1 -> Subtract_1063e/2
  Divide_dcd7a/1 -> Subtract_0afce/1
  Divide_b6dbe/1 -> Subtract_0afce/2
  State_E_fd_SG_D_3_2d5b6/1 -> Subtract_617ae/1
  State_psi_fd_SG_D_3_8c274/1 -> Subtract_617ae/2
  Subtract_1063e/1 -> Product_11951/1
  Subtract_617ae/1 -> Subtract_19629/1
  Product_11951/1 -> Subtract_19629/2
  Subtract_19629/1 -> Divide_27c8b/1
  Constant_T_dd_9c02c/1 -> Divide_27c8b/2
  Divide_27c8b/1 -> Blockout_d_psi_fd_SG_D_3_c1dbd/1

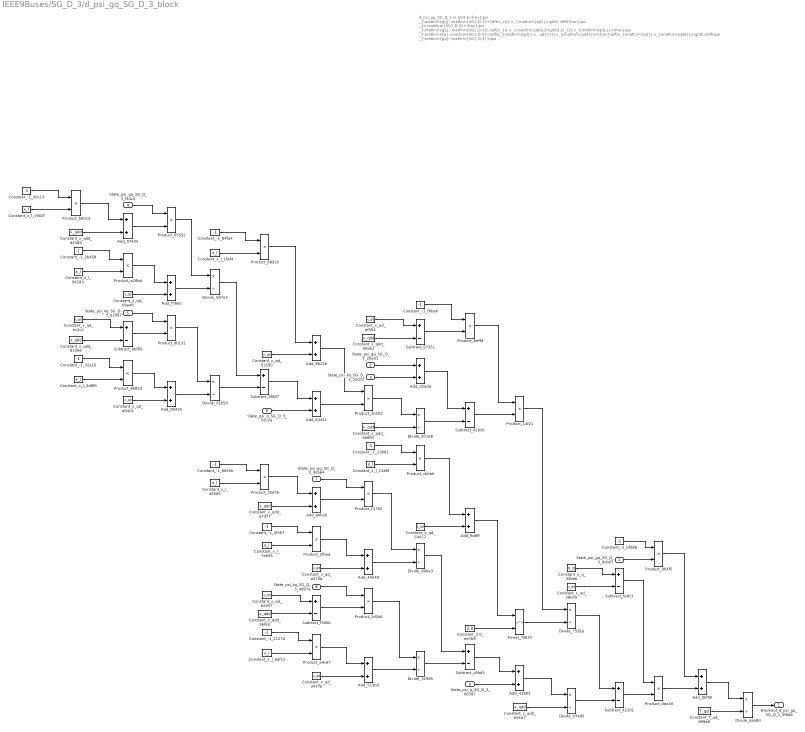
== system IEEE9Buses/SG_D_3/d_psi_gq_SG_D_3_block ==
  note: d_psi_gq_SG_D_3 in SG9
      | $-\frac{\psi _{\mathrm{gq},\mathrm{SG},D,3}+\left(x_{q}-x_{\mathrm{qd}}\right)\,\left(\frac{\psi _{q,\mathrm{SG},D,3}+\frac{\psi _{\mathrm{gq},\mathrm{SG},D,3}\,\left(x_{l}-x_{\mathrm{qdd}}\right)}{x_{l}-x_{\mathrm{qd}}}+\frac{\psi _{\mathrm{kq},\mathrm{SG},D,3}\,\left(x_{\mathrm{qd}}-x_{\mathrm{qdd}}\right)}{x_{l}-x_{\mathrm{qd}}}}{x_{\mathrm{qdd}}}+\frac{\left(x_{\mathrm{qd}}-x_{\mathrm{qdd}}\right)\,\left(\psi _{\mathrm{gq},\mathrm{SG},D,3}+\psi _{\mathrm{kq},\mathrm{SG},D,3}+\frac{\left(x_{l}-x_{\mathrm{qd}}\right)\,\left(\psi _{q,\mathrm{SG},D,3}+\frac{\psi _{\mathrm{gq},\mathrm{SG},D,3}\,\left(x_{l}-x_{\mathrm{qdd}}\right)}{x_{l}-x_{\mathrm{qd}}}+\frac{\psi _{\mathrm{kq},\mathrm{SG},D,3}\,\left(x_{\mathrm{qd}}-x_{\mathrm{qdd}}\right)}{x_{l}-x_{\mathrm{qd}}}\right)}{x_{\mathrm{qdd}}}\right)}{{\left(x_{l}-x_{\mathrm{qd}}\right)}^2}\right)}{T_{\mathrm{qd}}}$
      | Automatically generated on 2025-09-12 21:33:22 .
  State_psi_gq_SG_D_3_dcbd7 : Inport
  State_psi_gq_SG_D_3_25e31 : Inport  Port=2
  State_psi_kq_SG_D_3_22d72 : Inport  Port=3
  State_psi_gq_SG_D_3_f44c4 : Inport  Port=4
  State_psi_kq_SG_D_3_e1997 : Inport  Port=5
  State_psi_q_SG_D_3_5ec2a : Inport  Port=6
  State_psi_gq_SG_D_3_9c664 : Inport  Port=7
  State_psi_kq_SG_D_3_4d97e : Inport  Port=8
  State_psi_q_SG_D_3_66397 : Inport  Port=9
  Add_0bf90 : Sum
  Add_{41893,44249,64411,80425,97435} (5 alike) : Sum
  Add_513bd : Sum
  Add_8b22b : Sum
  Add_abb26 : Sum
  Add_d2add : Sum
  Add_f78eb : Sum
  Add_fbd9f : Sum
  Constant_-1_2127d : Constant  Value=-1
  Constant_-1_23082 : Constant  Value=-1
  Constant_-1_2b458 : Constant  Value=-1
  Constant_-1_32a16 : Constant  Value=-1
  Constant_-1_36c13 : Constant  Value=-1
  Constant_-1_4f367 : Constant  Value=-1
  Constant_-1_84fa4 : Constant  Value=-1
  Constant_-1_86e5b : Constant  Value=-1
  Constant_-1_bf086 : Constant  Value=-1
  Constant_-1_f6ba6 : Constant  Value=-1
  Constant_2.0_ee7b9 : Constant  Value=2.0
  Constant_T_qd_899a8 : Constant  Value=T_qd
  Constant_x_l_1faf4 : Constant  Value=x_l
  Constant_x_l_21a6f : Constant  Value=x_l
  Constant_x_l_46585 : Constant  Value=x_l
  Constant_x_l_5d8f0 : Constant  Value=x_l
  Constant_x_l_6df12 : Constant  Value=x_l
  Constant_x_l_7a656 : Constant  Value=x_l
  Constant_x_l_94183 : Constant  Value=x_l
  Constant_x_l_c902f : Constant  Value=x_l
  Constant_x_q_35beb : Constant  Value=x_q
  Constant_x_qd_28b7e : Constant  Value=x_qd
  Constant_x_qd_3477b : Constant  Value=x_qd
  Constant_x_qd_52590 : Constant  Value=x_qd
  Constant_x_qd_54017 : Constant  Value=x_qd
  Constant_x_qd_69a48 : Constant  Value=x_qd
  Constant_x_qd_a04c4 : Constant  Value=x_qd
  Constant_x_qd_a570a : Constant  Value=x_qd
  Constant_x_qd_af354 : Constant  Value=x_qd
  Constant_x_qd_b5057 : Constant  Value=x_qd
  Constant_x_qd_ec2c2 : Constant  Value=x_qd
  Constant_x_qdd_00ee1 : Constant  Value=x_qdd
  Constant_x_qdd_36fed : Constant  Value=x_qdd
  Constant_x_qdd_61266 : Constant  Value=x_qdd
  Constant_x_qdd_66893 : Constant  Value=x_qdd
  Constant_x_qdd_a7d77 : Constant  Value=x_qdd
  Constant_x_qdd_b91e7 : Constant  Value=x_qdd
  Constant_x_qdd_d43d9 : Constant  Value=x_qdd
  Divide_3195d : Product  Inputs=*/
  Divide_32965 : Product  Inputs=*/
  Divide_587e3 : Product  Inputs=*/
  Divide_7591e : Product  Inputs=*/
  Divide_800e3 : Product  Inputs=*/
  Divide_871e8 : Product  Inputs=*/
  Divide_d74d5 : Product  Inputs=*/
  Divide_daa8d : Product  Inputs=*/
  Power_fd625 : Math  Operator=pow
  Product_14f21 : Product
  Product_1d1b6 : Product
  Product_2b103 : Product
  Product_2fbea : Product
  Product_35d76 : Product
  Product_65592 : Product
  Product_68d10 : Product
  Product_6effd : Product
  Product_8681d : Product
  Product_a28bb : Product
  Product_b8015 : Product
  Product_c1762 : Product
  Product_cb0a6 : Product
  Product_d64f5 : Product
  Product_daa3d : Product
  Product_db131 : Product
  Product_e4c67 : Product
  Subtract_3f087 : Sum  Inputs=+-
  Subtract_41b30 : Sum  Inputs=+-
  Subtract_42101 : Sum  Inputs=+-
  Subtract_67351 : Sum  Inputs=+-
  Subtract_abfb5 : Sum  Inputs=+-
  Subtract_c8bd3 : Sum  Inputs=+-
  Subtract_f306b : Sum  Inputs=+-
  Subtract_fe8c3 : Sum  Inputs=+-
  Blockout_d_psi_gq_SG_D_3_5f8a8 : Outport
  wires:
  Constant_x_l_21a6f/1 -> Product_cb0a6/2
  Constant_x_qd_ec2c2/1 -> Subtract_abfb5/1
  Add_8b22b/1 -> Product_2b103/1
  Constant_-1_36c13/1 -> Product_b8015/1
  Add_97435/1 -> Product_65592/2
  Constant_x_qdd_61266/1 -> Subtract_abfb5/2
  Constant_x_qd_52590/1 -> Add_8b22b/2
  Constant_x_l_c902f/1 -> Product_b8015/2
  Constant_x_l_94183/1 -> Product_a28bb/2
  Add_513bd/1 -> Divide_32965/2
  State_psi_kq_SG_D_3_22d72/1 -> Add_d2add/2
  Constant_x_qdd_d43d9/1 -> Add_97435/2
  Product_b8015/1 -> Add_97435/1
  Constant_x_qd_3477b/1 -> Add_513bd/2
  Product_6effd/1 -> Product_14f21/1
  Constant_-1_86e5b/1 -> Product_35d76/1
  Constant_-1_2b458/1 -> Product_a28bb/1
  Constant_-1_32a16/1 -> Product_8681d/1
  Constant_x_l_5d8f0/1 -> Product_8681d/2
  Constant_-1_f6ba6/1 -> Product_6effd/1
  Constant_-1_bf086/1 -> Product_d64f5/1
  State_psi_gq_SG_D_3_f44c4/1 -> Product_65592/1
  Product_35d76/1 -> Add_abb26/1
  Product_a28bb/1 -> Add_f78eb/1
  Product_e4c67/1 -> Add_513bd/1
  Constant_x_qd_69a48/1 -> Add_f78eb/2
  Constant_-1_4f367/1 -> Product_2fbea/1
  State_psi_kq_SG_D_3_e1997/1 -> Product_db131/1
  Subtract_abfb5/1 -> Product_db131/2
  Product_8681d/1 -> Add_80425/1
  Add_abb26/1 -> Product_c1762/2
  Add_f78eb/1 -> Divide_587e3/2
  Constant_x_qd_a04c4/1 -> Add_80425/2
  Product_65592/1 -> Divide_587e3/1
  Constant_T_qd_899a8/1 -> Divide_daa8d/2
  Product_2fbea/1 -> Add_44249/1
  Product_db131/1 -> Divide_3195d/1
  Product_1d1b6/1 -> Divide_32965/1
  Add_80425/1 -> Divide_3195d/2
  Constant_-1_84fa4/1 -> Product_68d10/1
  Constant_x_qdd_66893/1 -> Divide_871e8/2
  Constant_x_l_1faf4/1 -> Product_68d10/2
  Divide_587e3/1 -> Subtract_3f087/1
  Constant_x_qd_28b7e/1 -> Subtract_fe8c3/2
  Add_44249/1 -> Divide_800e3/2
  Divide_3195d/1 -> Subtract_3f087/2
  Constant_x_l_46585/1 -> Product_35d76/2
  Product_68d10/1 -> Add_8b22b/1
  Constant_-1_23082/1 -> Product_cb0a6/1
  Constant_x_l_7a656/1 -> Product_2fbea/2
  Subtract_3f087/1 -> Add_64411/1
  State_psi_q_SG_D_3_5ec2a/1 -> Add_64411/2
  Constant_-1_2127d/1 -> Product_e4c67/1
  Constant_x_qdd_a7d77/1 -> Add_abb26/2
  Constant_x_qd_b5057/1 -> Subtract_f306b/1
  Constant_x_qdd_36fed/1 -> Subtract_f306b/2
  Constant_x_l_6df12/1 -> Product_e4c67/2
  Add_64411/1 -> Product_2b103/2
  Constant_x_qdd_00ee1/1 -> Subtract_67351/2
  State_psi_gq_SG_D_3_9c664/1 -> Product_c1762/1
  Constant_x_qd_a570a/1 -> Add_44249/2
  Divide_7591e/1 -> Subtract_42101/1
  State_psi_kq_SG_D_3_4d97e/1 -> Product_1d1b6/1
  Subtract_f306b/1 -> Product_1d1b6/2
  Constant_x_qd_af354/1 -> Subtract_67351/1
  State_psi_gq_SG_D_3_25e31/1 -> Add_d2add/1
  Product_2b103/1 -> Divide_871e8/1
  Product_c1762/1 -> Divide_800e3/1
  Subtract_67351/1 -> Product_6effd/2
  Add_d2add/1 -> Subtract_41b30/1
  Divide_871e8/1 -> Subtract_41b30/2
  Product_cb0a6/1 -> Add_fbd9f/1
  Constant_x_qd_54017/1 -> Add_fbd9f/2
  Divide_800e3/1 -> Subtract_c8bd3/1
  Divide_32965/1 -> Subtract_c8bd3/2
  Subtract_41b30/1 -> Product_14f21/2
  Add_fbd9f/1 -> Power_fd625/1
  Constant_2.0_ee7b9/1 -> Power_fd625/2
  Subtract_c8bd3/1 -> Add_41893/1
  State_psi_q_SG_D_3_66397/1 -> Add_41893/2
  Product_14f21/1 -> Divide_7591e/1
  Power_fd625/1 -> Divide_7591e/2
  Add_41893/1 -> Divide_d74d5/1
  Constant_x_qdd_b91e7/1 -> Divide_d74d5/2
  Constant_x_q_35beb/1 -> Subtract_fe8c3/1
  Divide_d74d5/1 -> Subtract_42101/2
  State_psi_gq_SG_D_3_dcbd7/1 -> Product_d64f5/2
  Subtract_fe8c3/1 -> Product_daa3d/1
  Subtract_42101/1 -> Product_daa3d/2
  Product_d64f5/1 -> Add_0bf90/1
  Product_daa3d/1 -> Add_0bf90/2
  Add_0bf90/1 -> Divide_daa8d/1
  Divide_daa8d/1 -> Blockout_d_psi_gq_SG_D_3_5f8a8/1

== system IEEE9Buses/SG_D_3/d_psi_kq_SG_D_3_block ==
  note: d_psi_kq_SG_D_3 in SG9
      | $-\frac{\psi _{\mathrm{gq},\mathrm{SG},D,3}+\psi _{\mathrm{kq},\mathrm{SG},D,3}+\frac{\left(x_{l}-x_{\mathrm{qd}}\right)\,\left(\psi _{q,\mathrm{SG},D,3}+\frac{\psi _{\mathrm{gq},\mathrm{SG},D,3}\,\left(x_{l}-x_{\mathrm{qdd}}\right)}{x_{l}-x_{\mathrm{qd}}}+\frac{\psi _{\mathrm{kq},\mathrm{SG},D,3}\,\left(x_{\mathrm{qd}}-x_{\mathrm{qdd}}\right)}{x_{l}-x_{\mathrm{qd}}}\right)}{x_{\mathrm{qdd}}}}{T_{\mathrm{qdd}}}$
      | Automatically generated on 2025-09-12 21:33:25 .
  State_psi_gq_SG_D_3_0b255 : Inport
  State_psi_kq_SG_D_3_9a42a : Inport  Port=2
  State_psi_gq_SG_D_3_70610 : Inport  Port=3
  State_psi_kq_SG_D_3_37576 : Inport  Port=4
  State_psi_q_SG_D_3_7d7d5 : Inport  Port=5
  Add_19248 : Sum
  Add_4037b : Sum
  Add_41302 : Sum
  Add_7c2a3 : Sum
  Add_a6a1b : Sum
  Add_b81ef : Sum
  Constant_-1_5c238 : Constant  Value=-1
  Constant_-1_65cd7 : Constant  Value=-1
  Constant_-1_9bbbf : Constant  Value=-1
  Constant_-1_cf6bd : Constant  Value=-1
  Constant_-1_ff1e3 : Constant  Value=-1
  Constant_T_qdd_c58b9 : Constant  Value=T_qdd
  Constant_x_l_070ca : Constant  Value=x_l
  Constant_x_l_15375 : Constant  Value=x_l
  Constant_x_l_441cb : Constant  Value=x_l
  Constant_x_l_87140 : Constant  Value=x_l
  Constant_x_qd_5176d : Constant  Value=x_qd
  Constant_x_qd_58580 : Constant  Value=x_qd
  Constant_x_qd_5ef40 : Constant  Value=x_qd
  Constant_x_qd_8b5ac : Constant  Value=x_qd
  Constant_x_qdd_2a781 : Constant  Value=x_qdd
  Constant_x_qdd_cbd82 : Constant  Value=x_qdd
  Constant_x_qdd_d65d4 : Constant  Value=x_qdd
  Divide_048d8 : Product  Inputs=*/
  Divide_1ffb7 : Product  Inputs=*/
  Divide_c43d5 : Product  Inputs=*/
  Divide_e69c3 : Product  Inputs=*/
  Product_3d7dc : Product
  Product_5759f : Product
  Product_85606 : Product
  Product_876e2 : Product
  Product_a1ba5 : Product
  Product_bab30 : Product
  Product_bfd1b : Product
  Product_ff6b1 : Product
  Subtract_6fb89 : Sum  Inputs=+-
  Subtract_77e4f : Sum  Inputs=+-
  Subtract_8f831 : Sum  Inputs=+-
  Blockout_d_psi_kq_SG_D_3_b0c25 : Outport
  wires:
  State_psi_q_SG_D_3_7d7d5/1 -> Add_a6a1b/2
  Constant_-1_5c238/1 -> Product_3d7dc/1
  Constant_-1_65cd7/1 -> Product_bfd1b/1
  Constant_-1_cf6bd/1 -> Product_85606/1
  Constant_x_l_15375/1 -> Product_3d7dc/2
  Constant_x_qdd_2a781/1 -> Add_b81ef/2
  Product_a1ba5/1 -> Add_41302/1
  Constant_x_l_070ca/1 -> Product_bfd1b/2
  Constant_x_qd_58580/1 -> Subtract_8f831/1
  Product_bfd1b/1 -> Add_b81ef/1
  Constant_x_l_87140/1 -> Product_876e2/2
  Constant_x_qdd_d65d4/1 -> Subtract_8f831/2
  Constant_-1_ff1e3/1 -> Product_a1ba5/1
  Constant_x_l_441cb/1 -> Product_a1ba5/2
  State_psi_gq_SG_D_3_70610/1 -> Product_5759f/1
  Add_b81ef/1 -> Product_5759f/2
  Add_a6a1b/1 -> Product_ff6b1/2
  Product_3d7dc/1 -> Add_19248/1
  Constant_x_qd_8b5ac/1 -> Add_19248/2
  State_psi_kq_SG_D_3_37576/1 -> Product_bab30/1
  Subtract_8f831/1 -> Product_bab30/2
  Add_19248/1 -> Divide_e69c3/2
  Constant_x_qd_5176d/1 -> Add_41302/2
  Product_5759f/1 -> Divide_e69c3/1
  Product_bab30/1 -> Divide_048d8/1
  Add_41302/1 -> Divide_048d8/2
  Constant_-1_9bbbf/1 -> Product_876e2/1
  Divide_e69c3/1 -> Subtract_77e4f/1
  Add_4037b/1 -> Divide_c43d5/1
  Divide_048d8/1 -> Subtract_77e4f/2
  Divide_c43d5/1 -> Blockout_d_psi_kq_SG_D_3_b0c25/1
  Product_876e2/1 -> Add_7c2a3/1
  Constant_x_qd_5ef40/1 -> Add_7c2a3/2
  Subtract_77e4f/1 -> Add_a6a1b/1
  State_psi_gq_SG_D_3_0b255/1 -> Product_85606/2
  Add_7c2a3/1 -> Product_ff6b1/1
  Constant_T_qdd_c58b9/1 -> Divide_c43d5/2
  Product_85606/1 -> Subtract_6fb89/1
  State_psi_kq_SG_D_3_9a42a/1 -> Subtract_6fb89/2
  Product_ff6b1/1 -> Divide_1ffb7/1
  Constant_x_qdd_cbd82/1 -> Divide_1ffb7/2
  Subtract_6fb89/1 -> Add_4037b/1
  Divide_1ffb7/1 -> Add_4037b/2

== system IEEE9Buses/SG_D_3/d_psi_q_SG_D_3_block ==
  note: d_psi_q_SG_D_3 in SG9
      | $2\,\pi \,f_{0}\,\left(v_{d,\mathrm{SG},D,3}\,\cos\left(\theta _{\mathrm{SG},D,3}\right)+v_{q,\mathrm{SG},D,3}\,\sin\left(\theta _{\mathrm{SG},D,3}\right)-\frac{R_{a}\,\left(\psi _{q,\mathrm{SG},D,3}+\frac{\psi _{\mathrm{gq},\mathrm{SG},D,3}\,\left(x_{l}-x_{\mathrm{qdd}}\right)}{x_{l}-x_{\mathrm{qd}}}+\frac{\psi _{\mathrm{kq},\mathrm{SG},D,3}\,\left(x_{\mathrm{qd}}-x_{\mathrm{qdd}}\right)}{x_{l}-x_{\mathrm{qd}}}\right)}{x_{\mathrm{qdd}}}-\frac{\psi _{d,\mathrm{SG},D,3}\,w_{\mathrm{SG},D,3}}{2\,f_{0}\,\pi }\right)$
      | Automatically generated on 2025-09-12 21:33:09 .
  State_psi_gq_SG_D_3_f88ed : Inport
  State_psi_kq_SG_D_3_b8c88 : Inport  Port=2
  State_psi_q_SG_D_3_144cc : Inport  Port=3
  Input_v_d_SG_D_3_fa4a6 : Inport  Port=4
  State_theta_SG_D_3_c2f12 : Inport  Port=5
  Input_v_q_SG_D_3_d1053 : Inport  Port=6
  State_theta_SG_D_3_c1394 : Inport  Port=7
  State_psi_d_SG_D_3_5ea0e : Inport  Port=8
  State_w_SG_D_3_05eca : Inport  Port=9
  Add_1724e : Sum
  Add_56afa : Sum
  Add_5d190 : Sum
  Add_a00de : Sum
  Add_b692e : Sum
  Constant_-1_337b3 : Constant  Value=-1
  Constant_-1_44d27 : Constant  Value=-1
  Constant_-1_9fee9 : Constant  Value=-1
  Constant_-2.0_d6a6c : Constant  Value=-2.0
  Constant_2.0_20e57 : Constant  Value=2.0
  Constant_R_a_b7d95 : Constant  Value=R_a
  Constant_f0_d6e13 : Constant  Value=f0
  Constant_f0_f9b96 : Constant  Value=f0
  Constant_pi_1159f : Constant  Value=pi
  Constant_pi_182f2 : Constant  Value=pi
  Constant_x_l_049e4 : Constant  Value=x_l
  Constant_x_l_3d785 : Constant  Value=x_l
  Constant_x_l_63f4a : Constant  Value=x_l
  Constant_x_qd_036fe : Constant  Value=x_qd
  Constant_x_qd_37600 : Constant  Value=x_qd
  Constant_x_qd_ed01e : Constant  Value=x_qd
  Constant_x_qdd_015a1 : Constant  Value=x_qdd
  Constant_x_qdd_16b3a : Constant  Value=x_qdd
  Constant_x_qdd_98b7d : Constant  Value=x_qdd
  Divide_238ee : Product  Inputs=*/
  Divide_3bafa : Product  Inputs=*/
  Divide_b830b : Product  Inputs=*/
  Divide_fbe14 : Product  Inputs=*/
  MathFunc_cos_72ab6 : Trigonometry  Operator=cos
  MathFunc_sin_eda63 : Trigonometry
  Product_06d27 : Product
  Product_246f0 : Product
  Product_4bdf0 : Product
  Product_7990c : Product
  Product_7f690 : Product
  Product_816ee : Product
  Product_8ce84 : Product
  Product_aa946 : Product
  Product_ade2c : Product
  Product_c8652 : Product
  Product_e12a0 : Product
  Product_e4fd6 : Product
  Product_efb59 : Product
  Product_ffeab : Product
  Subtract_023a6 : Sum  Inputs=+-
  Subtract_54955 : Sum  Inputs=+-
  Subtract_6734a : Sum  Inputs=+-
  Subtract_d2291 : Sum  Inputs=+-
  Blockout_d_psi_q_SG_D_3_07f24 : Outport
  wires:
  Constant_x_qd_036fe/1 -> Subtract_023a6/1
  Constant_pi_182f2/1 -> Product_7990c/2
  Product_ffeab/1 -> Divide_238ee/1
  Constant_x_l_3d785/1 -> Product_efb59/2
  Constant_f0_d6e13/1 -> Product_aa946/2
  State_w_SG_D_3_05eca/1 -> Product_8ce84/2
  Constant_-1_9fee9/1 -> Product_ade2c/1
  Constant_x_qdd_98b7d/1 -> Add_a00de/2
  Input_v_d_SG_D_3_fa4a6/1 -> Product_4bdf0/1
  Constant_x_qdd_16b3a/1 -> Subtract_023a6/2
  Constant_x_l_63f4a/1 -> Product_ade2c/2
  Divide_b830b/1 -> Add_b692e/2
  Product_ade2c/1 -> Add_a00de/1
  Constant_2.0_20e57/1 -> Product_7990c/1
  Add_5d190/1 -> Product_ffeab/2
  Constant_-1_44d27/1 -> Product_efb59/1
  Constant_x_qd_37600/1 -> Add_1724e/2
  Constant_-1_337b3/1 -> Product_246f0/1
  Subtract_6734a/1 -> Subtract_d2291/1
  Constant_x_l_049e4/1 -> Product_246f0/2
  Subtract_d2291/1 -> Add_b692e/1
  Constant_f0_f9b96/1 -> Product_816ee/2
  State_theta_SG_D_3_c1394/1 -> MathFunc_sin_eda63/1
  Constant_x_qd_ed01e/1 -> Add_56afa/2
  State_psi_gq_SG_D_3_f88ed/1 -> Product_e12a0/1
  Add_a00de/1 -> Product_e12a0/2
  Product_7990c/1 -> Product_816ee/1
  Product_efb59/1 -> Add_56afa/1
  State_psi_kq_SG_D_3_b8c88/1 -> Product_e4fd6/1
  Subtract_023a6/1 -> Product_e4fd6/2
  Product_246f0/1 -> Add_1724e/1
  MathFunc_sin_eda63/1 -> Product_c8652/2
  Product_e12a0/1 -> Divide_3bafa/1
  Product_816ee/1 -> Divide_b830b/2
  Add_56afa/1 -> Divide_3bafa/2
  Product_e4fd6/1 -> Divide_fbe14/1
  Add_1724e/1 -> Divide_fbe14/2
  Input_v_q_SG_D_3_d1053/1 -> Product_c8652/1
  Divide_3bafa/1 -> Subtract_54955/1
  Subtract_54955/1 -> Add_5d190/1
  Divide_fbe14/1 -> Subtract_54955/2
  Divide_238ee/1 -> Subtract_6734a/1
  State_psi_q_SG_D_3_144cc/1 -> Add_5d190/2
  Product_c8652/1 -> Subtract_d2291/2
  Constant_R_a_b7d95/1 -> Product_ffeab/1
  State_theta_SG_D_3_c2f12/1 -> MathFunc_cos_72ab6/1
  Constant_x_qdd_015a1/1 -> Divide_238ee/2
  MathFunc_cos_72ab6/1 -> Product_4bdf0/2
  Constant_-2.0_d6a6c/1 -> Product_06d27/1
  Product_4bdf0/1 -> Subtract_6734a/2
  State_psi_d_SG_D_3_5ea0e/1 -> Product_8ce84/1
  Constant_pi_1159f/1 -> Product_06d27/2
  Product_8ce84/1 -> Divide_b830b/1
  Product_06d27/1 -> Product_aa946/1
  Product_aa946/1 -> Product_7f690/1
  Add_b692e/1 -> Product_7f690/2
  Product_7f690/1 -> Blockout_d_psi_q_SG_D_3_07f24/1

== system IEEE9Buses/SG_D_3/d_theta_SG_D_3_block ==
  note: d_theta_SG_D_3 in SG9
      | $w_{\mathrm{SG},D,3}-2\,\pi \,f_{0}$
      | Automatically generated on 2025-09-12 21:33:32 .
  State_w_SG_D_3_9ea4f : Inport
  Add_820ba : Sum
  Constant_-2.0_71b6c : Constant  Value=-2.0
  Constant_f0_1bd3f : Constant  Value=f0
  Constant_pi_27584 : Constant  Value=pi
  Product_63492 : Product
  Product_ccb0e : Product
  Blockout_d_theta_SG_D_3_9d209 : Outport
  wires:
  Constant_-2.0_71b6c/1 -> Product_ccb0e/1
  Constant_pi_27584/1 -> Product_ccb0e/2
  State_w_SG_D_3_9ea4f/1 -> Add_820ba/2
  Product_ccb0e/1 -> Product_63492/1
  Constant_f0_1bd3f/1 -> Product_63492/2
  Product_63492/1 -> Add_820ba/1
  Add_820ba/1 -> Blockout_d_theta_SG_D_3_9d209/1
